simulink model "Narnia_model"  (R2023b)
settings: Solver=VariableStepAuto  StartTime=0.0  StopTime=inf  FixedStep=1  RelTol=1e-3  EnableMultiTasking=on
undefined symbols (not defined in the file): A, B, C, DiscIntNeverNeededParam, E, HeatLimit, ks, P, Tf, Ts
libraries: simulink x4, eeGeneralControl x1, slpidlib x1, rllib x1
settings Model: Creator=The MathWorks, Inc.  LastModifiedBy=hdt
settings SolverCC: AlgebraicLoopSolver=TrustRegion  MinimalZcImpactIntegration=on
settings DataIOCC: LimitDataPoints=on  SaveFormat=Array
settings OptimizationCC: ReuseModelBlockBuffer=off  LifeSpan=inf
settings DebuggingCC: UnconnectedInputMsg=warning  UnconnectedOutputMsg=warning  UnconnectedLineMsg=warning  SFUnexpectedBacktrackingDiag=warning  SFNoUnconditionalDefaultTransitionDiag=warning  SFExecutionAtInitializationDiag=none  ArithmeticOperatorsInVariantConditions=warning
settings HardwareCC: ProdBitPerPointer=32  ProdBitPerSizeT=32  ProdBitPerPtrDiffT=32  ProdLargestAtomicFloat=None  ProdIntDivRoundTo=Undefined  ProdEndianess=Unspecified  ProdWordSize=32  ProdHWDeviceType=32-bit Generic
settings ModelReferenceCC: EnableRefExpFcnMdlSchedulingChecks=on  PropagateSignalLabelsOutOfModel=off
settings SFSimCC: SimUseLocalCustomCode=off  CustomCodeUndefinedFunction=UseInterfaceOnly
settings RTWCC: RTWUseLocalCustomCode=off
settings CodeAppCC: StateflowObjectComments=on
settings GRTTargetCC: TargetLangStandard=C89/C90 (ANSI)
settings ConfigComp: CovMetricSettings=dw  CovSaveCumulativeToWorkspaceVar=on  CovSaveSingleToWorkspaceVar=on  CovExternalEMLEnable=off  CovSFcnEnable=off

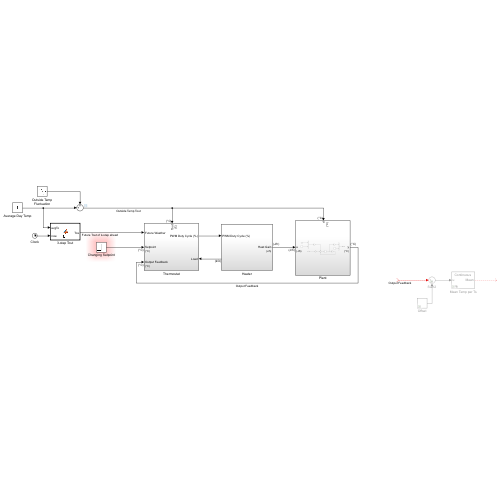
[thumbnail: Simulink's stored preview of the top-level diagram]
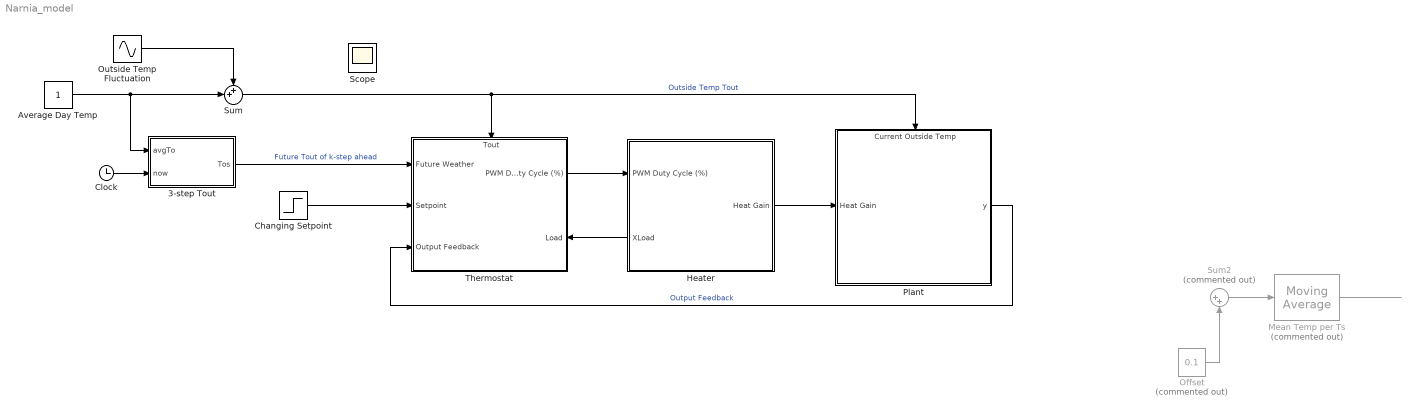
== system Narnia_model ==
  3-step Tout : MATLAB Function  TreatAsAtomicUnit=on
  Average Day Temp : Constant
  Changing Setpoint : Step  Time=Tf/2  Before=16.4102  After=17.7136  SampleTime=0  VectorParams1D=off
  Clock : Clock
  Heater : Subsystem
      settings: PortSchema="{\"entries\":[{\"content\":{\"sides\":[{\"content\":{\"connectorIds\":[\"In1\",\"Out2\"]},\"type\":\"ConnectorPlacement.EquallySpacedRectSide\",\"uuid\":\"4f8bdedb-4691-4645-9e5a-9d4cb9ebd4ea\"},{\"content\":{\"connectorIds\":[\"Out1\"],\"side\":\"RIGHT\"},\"type\":\"ConnectorPlacement.EquallySpacedRectSide\",\"uuid\":\"7d395606-f423-4b67-a102-5e58262706c1\"},{\"content\":{\"side\":\"TOP\"},\"type\":\"ConnectorPlacement.EquallySpacedRectSide\",\"uuid\":\"b7d096a7-af21-44a5-847f-d752d23dd21c\"}]},\"type\":\"ConnectorPlacement.EquallySpacedConnector\",\"uuid\":\"6f48db0c-acf9-47d8-b91b-c0b3a1fd4bfd\"}],\"packageUris\":[\"http://schema.mathworks.com/mf0/Connector/R2020b\"],\"version\":\"1.0\"}"
  Mean Temp per Ts : eeGeneralControl/Moving Average  Commented=on  VariantControl=Variant1  LabelModeActiveChoice=Continuous  f=1/Ts  x0=11  BufferSize=8192  Ts=0
      settings: LibrarySourceBlock=ee_sl_lib/General Control/Moving Average
  Offset : Constant  Commented=on  Value=0.1
  Outside Temp Fluctuation : Sin  Amplitude=4  Frequency=pi/12  SampleTime=0
  Plant : Subsystem
      settings: PortSchema="{\"entries\":[{\"content\":{\"sides\":[{\"content\":{\"connectorIds\":[\"In1\"]},\"type\":\"ConnectorPlacement.EquallySpacedRectSide\",\"uuid\":\"190832a2-0d7b-429a-8a42-d587dcc25890\"},{\"content\":{\"connectorIds\":[\"Out1\"],\"side\":\"RIGHT\"},\"type\":\"ConnectorPlacement.EquallySpacedRectSide\",\"uuid\":\"b8632c73-fea3-48b7-a581-c90e1ed24b24\"},{\"content\":{\"connectorIds\":[\"In2\"],\"side\":\"TOP\"},\"type\":\"ConnectorPlacement.EquallySpacedRectSide\",\"uuid\":\"193ecef7-bade-4674-8051-a43898fe5452\"}]},\"type\":\"ConnectorPlacement.EquallySpacedConnector\",\"uuid\":\"7b11e8d5-f5a5-413c-8c1c-b639b4d10c77\"}],\"packageUris\":[\"http://schema.mathworks.com/mf0/Connector/R2020b\"],\"version\":\"1.0\"}"
  Sum : Sum  Inputs=++|
  Sum2 : Sum  Commented=on  Inputs=|++
  Thermostat : Subsystem
      settings: PortSchema="{\"entries\":[{\"content\":{\"sides\":[{\"content\":{\"connectorIds\":[\"In1\",\"In2\",\"In3\"]},\"type\":\"ConnectorPlacement.EquallySpacedRectSide\",\"uuid\":\"895fbc35-389f-4678-9b0a-70c435693bfc\"},{\"content\":{\"connectorIds\":[\"Out1\",\"In5\"],\"side\":\"RIGHT\"},\"type\":\"ConnectorPlacement.EquallySpacedRectSide\",\"uuid\":\"8d167a41-533a-4be9-a4c1-965acf402f2c\"},{\"content\":{\"connectorIds\":[\"In4\"],\"side\":\"TOP\"},\"type\":\"ConnectorPlacement.EquallySpacedRectSide\",\"uuid\":\"c28d814a-5705-450e-be60-09afb29145b8\"},{\"content\":{\"side\":\"BOTTOM\"},\"type\":\"ConnectorPlacement.EquallySpacedRectSide\",\"uuid\":\"e32535bb-66ba-4e7f-9437-3af120630a67\"}]},\"type\":\"ConnectorPlacement.EquallySpacedConnector\",\"uuid\":\"9afdbd54-8878-403f-8397-85eadd1ad1fc\"}],\"packageUris\":[\"http://schema.mathworks.com/mf0/Connector/R2020b\"],\"version\":\"1.0\"}"
  Scope : Scope
  wires:
  Thermostat/1(PWM Duty Cycle (%)) -> Heater/1(PWM Duty Cycle (%))
  Heater/1(Heat Gain) -> Plant/1(Heat Gain)
  Plant/1(y) -> Thermostat/3(Output Feedback)  "Output Feedback"
  Heater/2(XLoad) -> Thermostat/5(Load)
  Clock/1 -> 3-step Tout/2(now)
  3-step Tout/1(Tos) -> Thermostat/1(Future Weather)  "Future Tout of k-step ahead"
  Average Day Temp/1 -> Sum/2, 3-step Tout/1(avgTo)
  Outside Temp Fluctuation/1 -> Sum/1
  Sum/1 -> Plant/2(Current Outside Temp), Thermostat/4(Tout)  "Outside Temp Tout"
  Changing Setpoint/1 -> Thermostat/2(Setpoint)
  ? -> Sum2/1  "Output Feedback"
  Offset/1 -> Sum2/2
  Sum2/1 -> Mean Temp per Ts/1
  Mean Temp per Ts/1 -> ?

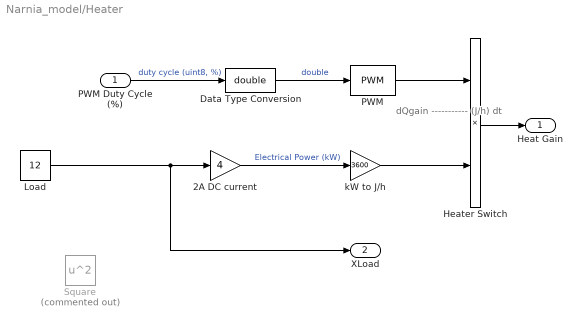
== system Narnia_model/Heater ==
  note: dQgain
      | ----------- (J/h)
      |    dt
  PWM Duty Cycle (%) : Inport
  2A DC current : Gain  Gain=4
  Data Type Conversion : DataTypeConversion  OutDataTypeStr=double  RndMeth=Round  SaturateOnIntegerOverflow=off
  Heater Switch : Product  RndMeth=Zero
  Load : Constant  Value=12
  PWM : simulink/Discontinuities/PWM  DisableCoverage=on  Period=P  InitialDelay=0  DisallowZeroDutyCycle=off  RunAtFixedTimeIntervals=off  SampleTime=0.1
  Square : Math  Commented=on  Operator=square
  kW to J/h : Gain  Gain=3600
  Heat Gain : Outport  Unit=joule/hour  VectorParamsAs1DForOutWhenUnconnected=off
  XLoad : Outport  Port=2  Unit=kΩ
  wires:
  PWM/1 -> Heater Switch/1
  Heater Switch/1 -> Heat Gain/1
  kW to J/h/1 -> Heater Switch/2
  PWM Duty Cycle (%)/1 -> Data Type Conversion/1  "duty cycle (uint8, %)"
  2A DC current/1 -> kW to J/h/1  "Electrical Power (kW)"
  Load/1 -> XLoad/1, 2A DC current/1
  Data Type Conversion/1 -> PWM/1  "double"

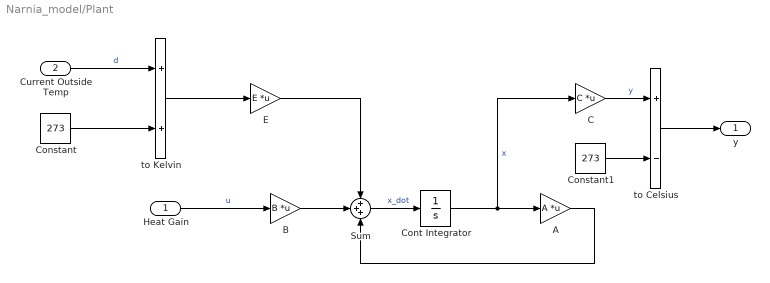
== system Narnia_model/Plant ==
  Heat Gain : Inport  Unit=J/h
  Current Outside Temp : Inport  Port=2  Unit=Celsius
  A : Gain  Gain=A  Multiplication=Matrix(K*u)
  B : Gain  Gain=B  Multiplication=Matrix(K*u)
  C : Gain  Gain=C  Multiplication=Matrix(K*u)
  Constant : Constant  Value=273
  Constant1 : Constant  Value=273
  Cont Integrator : Integrator  InitialCondition=289.3746
  E : Gain  Gain=E  Multiplication=Matrix(K*u)
  Sum : Sum  Inputs=+++
  to Celsius : Sum  Inputs=+-
  to Kelvin : Sum
  y : Outport  Unit=°C
  wires:
  Heat Gain/1 -> B/1  "u"
  B/1 -> Sum/2
  A/1 -> Sum/3
  Sum/1 -> Cont Integrator/1  "x_dot"
  Cont Integrator/1 -> C/1, A/1  "x"
  E/1 -> Sum/1
  Current Outside Temp/1 -> to Kelvin/1  "d"
  C/1 -> to Celsius/1  "y"
  Constant/1 -> to Kelvin/2
  to Kelvin/1 -> E/1
  to Celsius/1 -> y/1
  Constant1/1 -> to Celsius/2

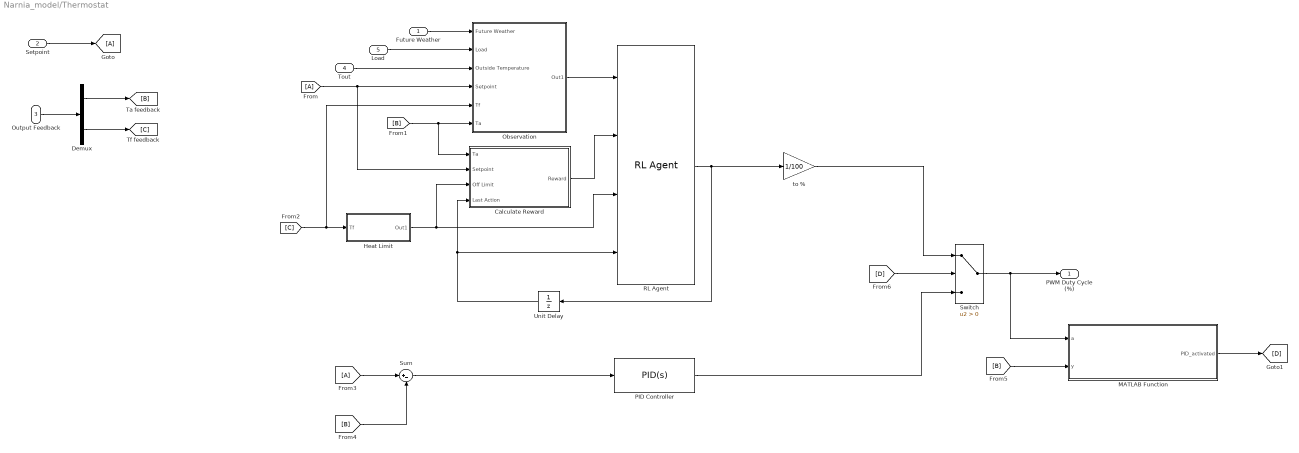
== system Narnia_model/Thermostat ==
  Future Weather : Inport
  Setpoint : Inport  Port=2  Unit=°C
  Output Feedback : Inport  Port=3  Unit=°C
  Tout : Inport  Port=4  Unit=°C
  Load : Inport  Port=5
  Calculate Reward : Subsystem
  Demux : Demux  Outputs=2
  From : From
  From3 : From
  Goto : Goto
  Heat Limit : Subsystem
  MATLAB Function : MATLAB Function  TreatAsAtomicUnit=on
  Observation : Subsystem
  PID Controller : slpidlib/PID Controller  Controller=PID  Form=Parallel  TimeDomain=Continuous-time  UseExternalTs=off  SampleTime=-1  IntegratorMethod=Forward Euler  FilterMethod=Forward Euler  ControllerParametersSource=internal  P=1  I=1  UseKiTs=off  D=0  N=100  UseFilter=on  TunerSelectOption=Transfer Function Based (PID Tuner App)  InitialConditionSource=internal  InitialConditionForIntegrator=0  InitialConditionForFilter=0  DifferentiatorICPrevScaledInput=0  ExternalReset=none  TrackingMode=off  Kt=1  LimitOutput=off  SatLimitsSource=internal  UpperSaturationLimit=inf  LowerSaturationLimit=-inf  LinearizeAsGain=on  AntiWindupMode=none  Kb=1  LimitIntegrator=off  UpperIntegratorSaturationLimit=inf  LowerIntegratorSaturationLimit=-inf  POutMin=[]  POutMax=[]  IOutMin=[]  IOutMax=[]  DOutMin=[]  DOutMax=[]  NOutMin=[]  NOutMax=[]  SumOutMin=[]  SumOutMax=[]  SaturationOutMin=[]  SaturationOutMax=[]  PParamMin=[]  PParamMax=[]  IParamMin=[]  IParamMax=[]  DParamMin=[]  DParamMax=[]  NParamMin=[]  NParamMax=[]  KbParamMin=[]  KbParamMax=[]  KtParamMin=[]  KtParamMax=[]  KbOutMin=[]  KbOutMax=[]  KtOutMin=[]  KtOutMax=[]  IntegratorOutMin=[]  IntegratorOutMax=[]  FilterOutMin=[]  FilterOutMax=[]  SumI1OutMin=[]  SumI1OutMax=[]  SumI2OutMin=[]  SumI2OutMax=[]  SumI3OutMin=[]  SumI3OutMax=[]  SumI4OutMin=[]  SumI4OutMax=[]  SumDOutMin=[]  SumDOutMax=[]  DifferentiatorOutMin=[]  DifferentiatorOutMax=[]  FilterDiffOutCoefMin=[]  FilterDiffOutCoefMax=[]  ReciprocalOutMin=[]  ReciprocalOutMax=[]  SumDenOutMin=[]  SumDenOutMax=[]  SumNumOutMin=[]  SumNumOutMax=[]  DivideOutMin=[]  DivideOutMax=[]  UdiffTsProdOutMin=[]  UdiffTsProdOutMax=[]  NTsProdOutMin=[]  NTsProdOutMax=[]  UintegralTsProdOutMin=[]  UintegralTsProdOutMax=[]  UngainTsProdOutMin=[]  UngainTsProdOutMax=[]  ClampingZeroOutDataTypeStr=Inherit: Inherit via back propagation  ClampingZeroOutMin=[]  ClampingZeroOutMax=[]  FilterDenConstantOutDataTypeStr=Inherit: Inherit via back propagation  FilterDenConstantOutMin=[]  FilterDenConstantOutMax=[]  PCopyOutDataTypeStr=Inherit: Inherit via back propagation  PCopyOutMin=[]  PCopyOutMax=[]  NCopyOutDataTypeStr=Inherit: Inherit via back propagation  NCopyOutMin=[]  NCopyOutMax=[]  IntegratorContinuousStateAttributes=''  IntegratorStateMustResolveToSignalObject=off  IntegratorRTWStateStorageClass=Auto  FilterContinuousStateAttributes=''  FilterStateMustResolveToSignalObject=off  FilterRTWStateStorageClass=Auto  ParallelPVariant=InternalParameters  IdealPVariant=Disabled  IVariant=InternalParameters  DVariant=InternalParameters  IntegratorVariant=Continuous  SatVariant=Disabled  AWVariant=Passthrough  PCopyVariant=Disabled  TRVariant=Disabled  FdbkBlocksVariant=Forward  IdealPFdbkVariant=Disabled  SatFdbkVariant=Disabled  DerivativeFilterVariant=ContFilter  NVariant=InternalParameters  NCopyVariant=Disabled  FilterICVariant=InternalICsFilter  IntegratorICVariant=InternalICs  ExternalResetVariant=Disabled  TRSumVariant=Passthrough  SumFdbkVariant=Disabled  SumVariant=Sum_PID  TsampFilterVariant=InternalTs  TsampNgainVariant=Passthrough  TsampIntegralVariant=Passthrough  ExternalSaturationOutDataTypeStr=Inherit: Same as second input
  RL Agent : rllib/RL Agent  Agent=default_agent  ExternalActionAsInput=off  ProvideLastAction=on  ProvideCumRwd=off  TreatAsDirectFeedthrough=on  UseStrictObservationDataTypes=off
  Sum : Sum  Inputs=|+-
  Switch : Switch  Criteria=u2 > Threshold  SaturateOnIntegerOverflow=off  InputSameDT=off
  Unit Delay : UnitDelay  SampleTime=-1  HasFrameUpgradeWarning=on
  to % : Gain  Gain=1/100
  PWM Duty Cycle (%) : Outport  VectorParamsAs1DForOutWhenUnconnected=off
  wires:
  From/1 -> Observation/4(Setpoint), Calculate Reward/2(Setpoint)
  [B] -> Calculate Reward/1(Ta), Observation/6(Ta)
  Tout/1 -> Observation/3(Outside Temperature)
  Observation/1(Out1) -> RL Agent/1
  Calculate Reward/1(Reward) -> RL Agent/2
  Heat Limit/1(Out1) -> Calculate Reward/3(Off Limit), RL Agent/3
  RL Agent/1 -> to %/1, Unit Delay/1
  Unit Delay/1 -> Calculate Reward/4(Last Action), RL Agent/4
  Load/1 -> Observation/2(Load)
  Future Weather/1 -> Observation/1(Future Weather)
  to %/1 -> Switch/1
  Setpoint/1 -> Goto/1
  Output Feedback/1 -> Demux/1
  Demux/1 -> [B]
  Demux/2 -> [C]
  [C] -> Observation/5(Tf), Heat Limit/1(Tf)
  From3/1 -> Sum/1
  [B] -> Sum/2
  Sum/1 -> PID Controller/1
  [B] -> MATLAB Function/2(y)
  Switch/1 -> PWM Duty Cycle (%)/1, MATLAB Function/1(a)
  PID Controller/1 -> Switch/3
  MATLAB Function/1(PID_activated) -> [D]
  [D] -> Switch/2

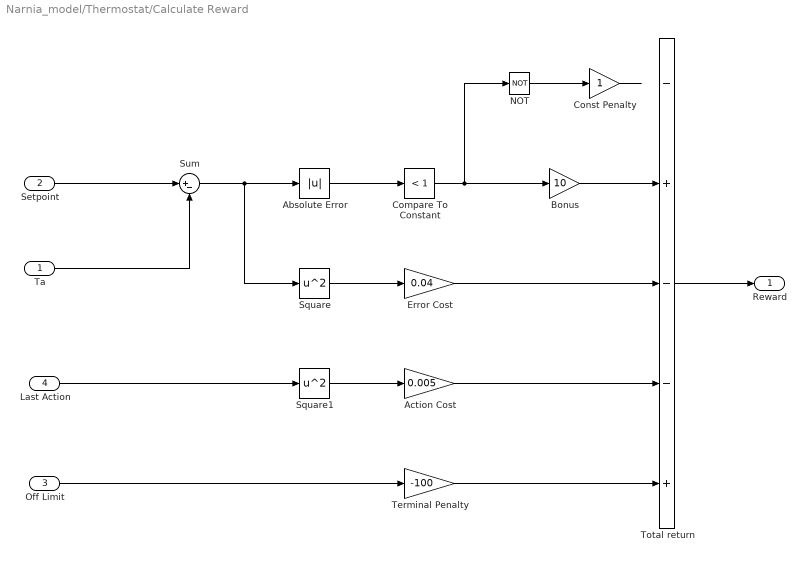
== system Narnia_model/Thermostat/Calculate Reward ==
  Ta : Inport
  Setpoint : Inport  Port=2
  Off Limit : Inport  Port=3
  Last Action : Inport  Port=4
  Absolute Error : Abs  SaturateOnIntegerOverflow=off
  Action Cost : Gain  Gain=0.005
  Bonus : Gain  Gain=10
  Compare To Constant : simulink/Logic and Bit Operations/Compare To Constant  relop=<  const=1  OutDataTypeStr=boolean
  Const Penalty : Gain
  Error Cost : Gain  Gain=0.04
  NOT : Logic  Operator=NOT  IconShape=distinctive  AllPortsSameDT=off  OutDataTypeStr=boolean
  Square : Math  Operator=square
  Square1 : Math  Operator=square
  Sum : Sum  Inputs=|+-
  Terminal Penalty : Gain  Gain=-100
  Total return : Sum  Inputs=-+--+
  Reward : Outport
  wires:
  Setpoint/1 -> Sum/1
  Total return/1 -> Reward/1
  Terminal Penalty/1 -> Total return/5
  Off Limit/1 -> Terminal Penalty/1
  Sum/1 -> Square/1, Absolute Error/1
  Absolute Error/1 -> Compare To Constant/1
  Bonus/1 -> Total return/2
  Compare To Constant/1 -> NOT/1, Bonus/1
  Const Penalty/1 -> ?
  NOT/1 -> Const Penalty/1
  Error Cost/1 -> Total return/3
  Square/1 -> Error Cost/1
  Square1/1 -> Action Cost/1
  Action Cost/1 -> Total return/4
  Last Action/1 -> Square1/1
  Ta/1 -> Sum/2

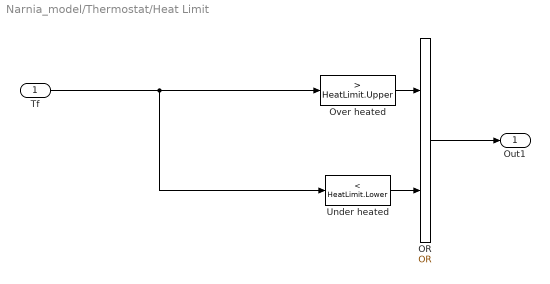
== system Narnia_model/Thermostat/Heat Limit ==
  Tf : Inport
  OR : Logic  Operator=OR  IconShape=distinctive  AllPortsSameDT=off  OutDataTypeStr=boolean
  Over heated : simulink/Logic and Bit Operations/Compare To Constant  relop=>  const=HeatLimit.Upper  OutDataTypeStr=boolean
  Under heated : simulink/Logic and Bit Operations/Compare To Constant  relop=<  const=HeatLimit.Lower  OutDataTypeStr=boolean
  Out1 : Outport
  wires:
  Under heated/1 -> OR/2
  Over heated/1 -> OR/1
  OR/1 -> Out1/1
  Tf/1 -> Under heated/1, Over heated/1

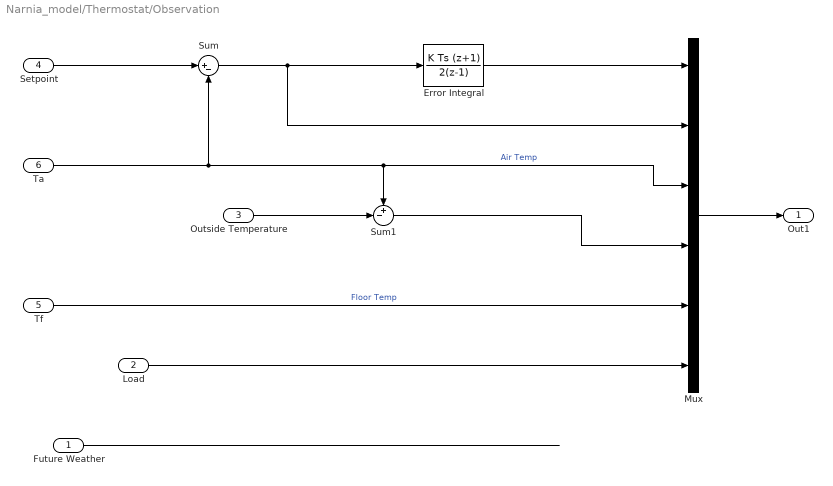
== system Narnia_model/Thermostat/Observation ==
  Future Weather : Inport
  Load : Inport  Port=2
  Outside Temperature : Inport  Port=3
  Setpoint : Inport  Port=4
  Tf : Inport  Port=5
  Ta : Inport  Port=6
  Error Integral : DiscreteIntegrator  IntegratorMethod=Integration: Trapezoidal  SampleTime=-1  ICPrevOutput=DiscIntNeverNeededParam  ICPrevScaledInput=DiscIntNeverNeededParam
  Mux : Mux  Inputs=6
  Sum : Sum  Inputs=|+-
  Sum1 : Sum  Inputs=+-|
  Out1 : Outport
  wires:
  Setpoint/1 -> Sum/1
  Ta/1 -> Sum/2, Sum1/1, Mux/3  "Air Temp"
  Error Integral/1 -> Mux/1
  Mux/1 -> Out1/1
  Sum/1 -> Error Integral/1, Mux/2
  Tf/1 -> Mux/5  "Floor Temp"
  Load/1 -> Mux/6
  Sum1/1 -> Mux/4
  Outside Temperature/1 -> Sum1/2
  Future Weather/1 -> ?

== matlab function Narnia_model/Thermostat/MATLAB Function ==
  data: a input; PID_activated output; y input
function PID_activated = activate_PID(a, y)
    % Generate residual
    r = a + y;
    % Make decision
PID_activated = (r >= 0);

== matlab function Narnia_model/3-step Tout ==
  settings: updateMethod=DISCRETE  sampleTime=Ts
  data: avgTo input; now input; Tos output size=horizon; ks parameter; Ts parameter
function Tos = fcn(avgTo, now, ks, Ts)
    Tos = 4*sin(pi/12 .* (now + ks*Ts) + 0) + avgTo;
end
